simulink subsystem "MMGHardware"  (R2023b)
settings: Solver=VariableStepAuto  StartTime=0.0  StopTime=10.0  RelTol=1e-3
settings Model: Creator=jaime  LastModifiedBy=jaime

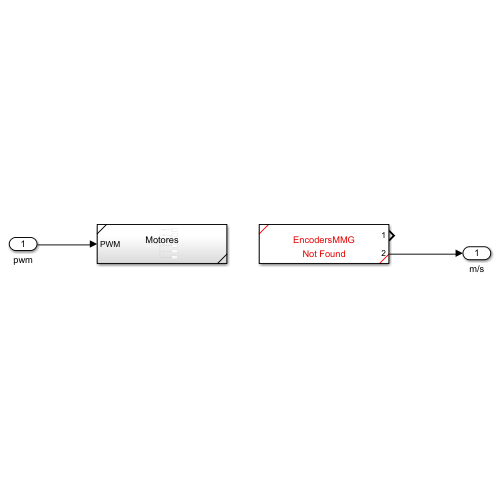
[thumbnail: Simulink's stored preview of the top-level diagram]
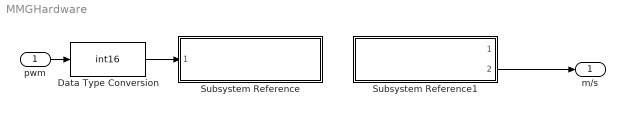
== system MMGHardware ==
  pwm : Inport
  Data Type Conversion : DataTypeConversion  OutDataTypeStr=int16  SaturateOnIntegerOverflow=off  RndMeth=Floor
  Subsystem Reference : Subsystem  ReferencedSubsystem=Motores
  Subsystem Reference1 : Subsystem  ReferencedSubsystem=EncodersAJ
  m/s : Outport
  wires:
  Subsystem Reference1/2 -> m/s/1
  pwm/1 -> Data Type Conversion/1
  Data Type Conversion/1 -> Subsystem Reference/1
